simulink model "Ejercicio2"  (R2015b)
settings: Solver=VariableStepAuto  StartTime=0.0  StopTime=0.1  MaxStep=0.001  RelTol=1e-3
settings Model: Creator=ariel  LastModifiedBy=ariel

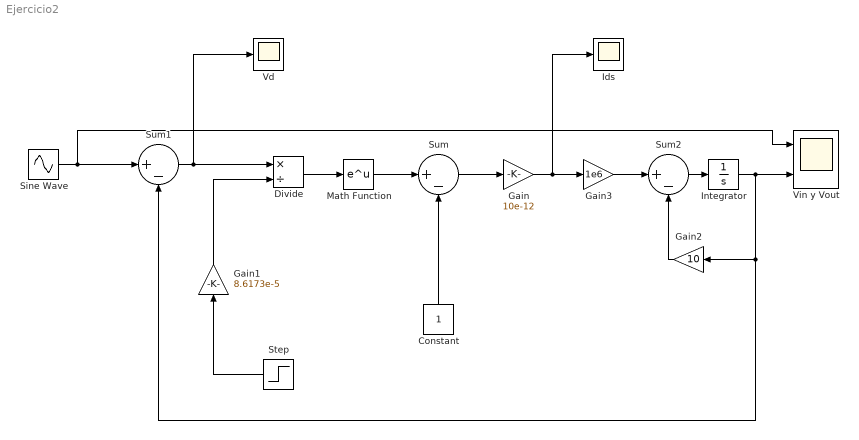
== system Ejercicio2 ==
  Constant : Constant
  Divide : Product  Inputs=*/
  Gain : Gain  Gain=10e-12
  Gain1 : Gain  Gain=8.6173e-5
  Gain2 : Gain  Gain=10
  Gain3 : Gain  Gain=1e6
  Ids : Scope
  Integrator : Integrator
  Math Function : Math  SaturateOnIntegerOverflow=on
  Sine Wave : Sin  Amplitude=12  Frequency=2*pi*60  SampleTime=0
  Step : Step  Time=0  After=300  SampleTime=0
  Sum : Sum  Inputs=|+-
  Sum1 : Sum  Inputs=|+-
  Sum2 : Sum  Inputs=|+-
  Vd : Scope
  Vin y Vout : Scope  NumInputPorts=2
  wires:
  Math Function/1 -> Sum/1
  Divide/1 -> Math Function/1
  Gain1/1 -> Divide/2
  Step/1 -> Gain1/1
  Sum1/1 -> Vd/1, Divide/1
  Sine Wave/1 -> Vin y Vout/1, Sum1/1
  Sum2/1 -> Integrator/1
  Gain/1 -> Ids/1, Gain3/1
  Constant/1 -> Sum/2
  Integrator/1 -> Vin y Vout/2, Gain2/1, Sum1/2
  Gain2/1 -> Sum2/2
  Sum/1 -> Gain/1
  Gain3/1 -> Sum2/1
